simulink library "wnnutils"  (R2021b)
settings: Solver=VariableStepAuto  StartTime=0.0  StopTime=10.0  RelTol=1e-3
settings Model: Creator=20214358  LastModifiedBy=20214358

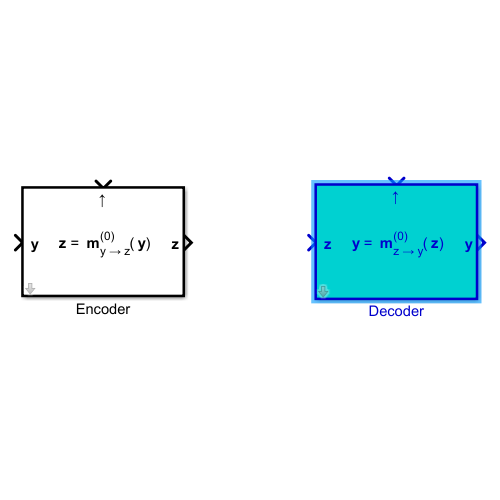
[thumbnail: Simulink's stored preview of the top-level diagram]
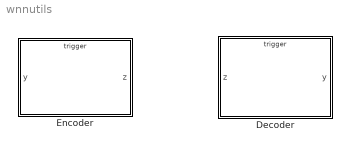
== system wnnutils ==
  Decoder : Subsystem  TreatAsAtomicUnit=on  mask{encoder_id=0, output_dims=2}
      mask prompts: encoder_id "Encoder id"; output_dims "Output dimensions"
      mask Display:
      | disp('{\bf y} = {\bf m}_{z \rightarrow y}^{(' + string(get_param(gcb, 'encoder_id'))+ ')}({\bf z})','interpreter','tex');
      | port_label('input', 1,'{\bf z}','interpreter','tex')
      | port_label('output', 1,'{\bf y}','interpreter','tex')
      | port_label('trigger','\uparrow','interpreter','tex')
  Encoder : Subsystem  mask{encoder_id=0, max_depth=16, learning_rate=0.001, min_splitting_volume=0.01, min_bounds=[0 0], max_bounds=[10 10]}
      mask prompts: encoder_id "Encoder id"; max_depth "Maximum depth"; learning_rate "Learning rate"; min_splitting_volume "Minimum splitting volume"; min_bounds "Minimum bounds"; max_bounds "Maximum bounds"
      mask Display:
      | disp('{\bf z} = {\bf m}_{y \rightarrow z}^{(' + string(get_param(gcb, 'encoder_id'))+ ')}({\bf y})','interpreter','tex');
      | port_label('input', 1,'{\bf y}','interpreter','tex')
      | port_label('output', 1,'{\bf z}','interpreter','tex')
      | port_label('trigger','\uparrow','interpreter','tex')

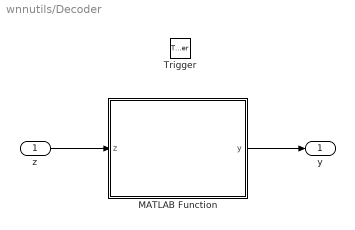
== system wnnutils/Decoder ==
  z : Inport
  Trigger : TriggerPort  VariantControl=(inherit)
  MATLAB Function : MATLAB Function  TreatAsAtomicUnit=on
  y : Outport
  wires:
  z/1 -> MATLAB Function/1(z)
  MATLAB Function/1(y) -> y/1

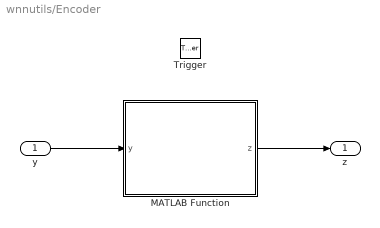
== system wnnutils/Encoder ==
  y : Inport
  Trigger : TriggerPort  VariantControl=(inherit)  OutputDataType=int8  InitialTriggerSignalState=zero  PortDimensions=1
  MATLAB Function : MATLAB Function  TreatAsAtomicUnit=on
  z : Outport
  wires:
  y/1 -> MATLAB Function/1(y)
  MATLAB Function/1(z) -> z/1

== matlab function wnnutils/Decoder/MATLAB Function ==
  data: z input; y output; encoder_id parameter; output_dims parameter
function y  = fcn(z, encoder_id, output_dims)

coder.extrinsic('py.wnnlib.decode');

y = zeros(1,output_dims,'double');
y = double(py.wnnlib.decode(encoder_id, uint8(z)));

== matlab function wnnutils/Encoder/MATLAB Function ==
  data: y input; encoder_id parameter; z output; max_depth parameter; learning_rate parameter; min_splitting_volume parameter; max_bounds parameter; min_bounds parameter
function z = fcn(y, encoder_id, max_depth, learning_rate, min_splitting_volume, max_bounds, min_bounds)

coder.extrinsic('py.wnnlib.add_encoder', 'py.wnnlib.encode');

persistent flag

if isempty(flag)
    py.wnnlib.add_encoder(encoder_id, max_depth, learning_rate, min_splitting_volume, min_bounds, max_bounds);
    flag = true;
end

z = zeros(1,max_depth,'logical');
z = logical(py.wnnlib.encode(encoder_id, y));
